simulink model "lab1b"  (R2023a)
settings: Solver=FixedStepAuto  StartTime=0.0  StopTime=1.0  FixedStep=1/(8*512)  RelTol=1e-3
settings Model: Creator=simja  LastModifiedBy=a96an
settings SolverCC: AutoInsertRateTranBlk=on
settings DataIOCC: ReturnWorkspaceOutputs=off
settings OptimizationCC: ReuseModelBlockBuffer=off

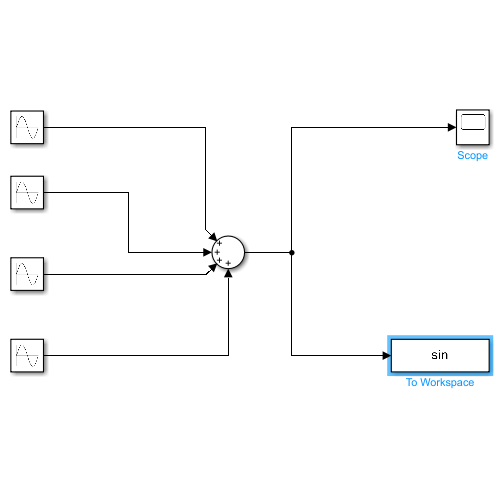
[thumbnail: Simulink's stored preview of the top-level diagram]
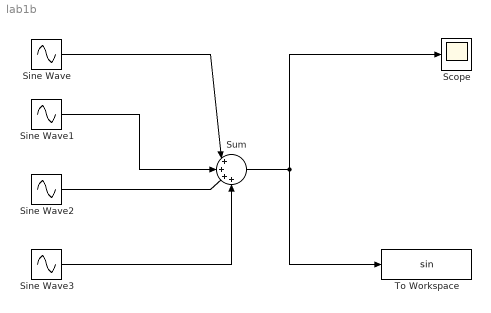
== system lab1b ==
  Scope : Scope
  Sine Wave : Sin  Amplitude=0.1  Frequency=2*pi*7  SampleTime=0
  Sine Wave1 : Sin  Amplitude=0.1  Frequency=2*pi*18  SampleTime=0
  Sine Wave2 : Sin  Amplitude=0.1  Frequency=2*pi*46  Phase=pi  SampleTime=0
  Sine Wave3 : Sin  Amplitude=0.1  Frequency=2*pi*65  SampleTime=0
  Sum : Sum  Inputs=|++++
  To Workspace : ToWorkspace  VariableName=sin  SaveFormat=Structure With Time  SampleTime=-1
  wires:
  Sine Wave3/1 -> Sum/4
  Sine Wave2/1 -> Sum/3
  Sine Wave1/1 -> Sum/2
  Sine Wave/1 -> Sum/1
  Sum/1 -> Scope/1, To Workspace/1
